simulink model "sampleModel196"  (R2021b)
settings: Solver=VariableStepAuto  StartTime=0.0  StopTime=10.0  RelTol=1e-3
undefined symbols (not defined in the file or in its folder): DiscIntNeverNeededParam
libraries: simulink x12, slpidlib x1
settings Model: Creator=user  LastModifiedBy=user

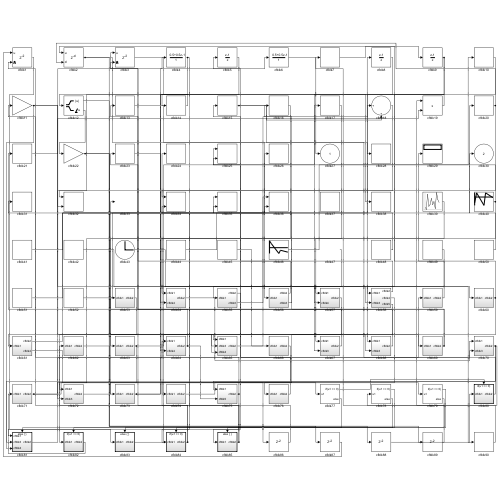
[thumbnail: Simulink's stored preview of the top-level diagram]
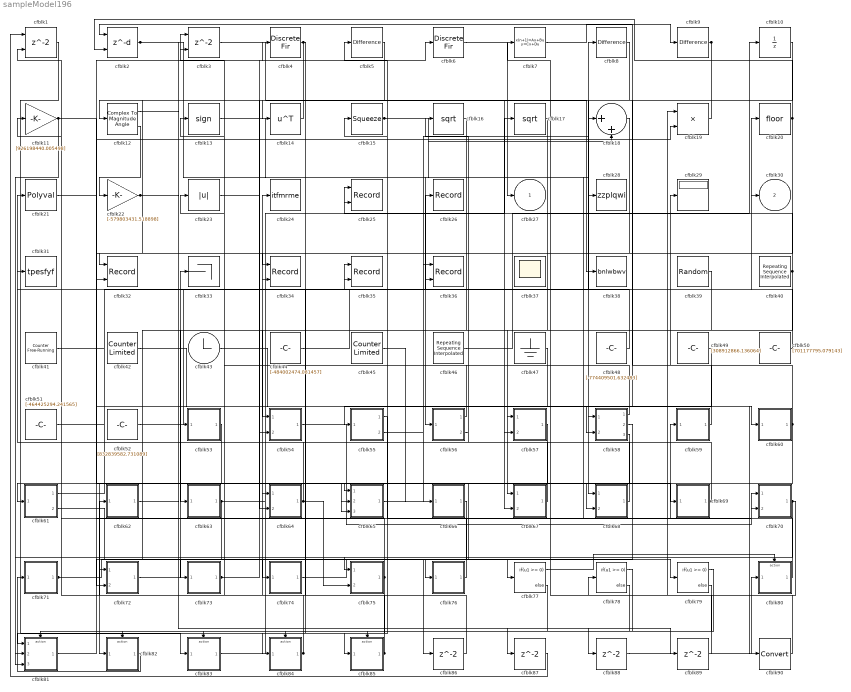
== system sampleModel196 ==
  cfblk1 : Delay  ShowEnablePort=on  SampleTime=1
      settings: InputPortMap=u0,e6
  cfblk10 : UnitDelay  HasFrameUpgradeWarning=on
  cfblk11 : Gain  Gain=[926198440.005498]
  cfblk12 : ComplexToMagnitudeAngle
  cfblk13 : Signum
  cfblk14 : Math  Operator=transpose  SaturateOnIntegerOverflow=on
  cfblk15 : Squeeze
  cfblk16 : Sqrt  SaturateOnIntegerOverflow=on
  cfblk17 : Sqrt  SaturateOnIntegerOverflow=on
  cfblk18 : Sum  Inputs=|++
  cfblk19 : Product  Inputs=**
  cfblk2 : Delay  DelayLengthSource=Input port  SampleTime=1
      settings: InputPortMap=u0,p1
  cfblk20 : Rounding
  cfblk21 : Polyval  Coefs=[ +2.081618890e-019, -1.441693666e-014, +4.719686976e-010, -8.536869453e-006, +1.621573104e-001, -8.087801117e+001 ]
  cfblk22 : Gain  Gain=[-579803431.518898]
  cfblk23 : Abs
  cfblk24 : ToWorkspace  VariableName=itfmrme  SaveFormat=Timeseries  SampleTime=-1
  cfblk25 : Record  FileSettingsInternal="{\"entries\":[{\"content\":{\"excelSettings\":{\"content\":{},\"type\":\"Streamout.ExcelSettings\"}},\"type\":\"Streamout.FileSettingStorage\",\"uuid\":\"ebd6f4a9-3581-428a-b59a-ad7a62004bd4\"}],\"packageUris\":[\"http://schema.mathworks.com/mf0/streamout_blocks/R2020a\"],\"version\":\"1.0\"}"  Layout=[1 1]  SignalsInternal="{\"entries\":[{\"content\":{\"signals\":[{\"content\":{\"blockPath\":[\"sampleModel196/cfblk25\"],\"channel\":[],\"dimensions\":[1],\"domain\":\"sampleModel196/cfblk25\",\"lineColor\":\"#a2142f\",\"plots\":[1],\"port\":1,\"sid\":[\"\"],\"signalID\":7449,\"signalName\":\"cfblk56:1\"},\"type\":\"RecordBlkView.Signal\",\"uuid\":\"a9c48982-f614-47e9-af30-97d896957ff6\"},{\"content\":{\"blockPath\":[\"sampleModel196/cfblk25\"],\"channel\":[],\"dimensions\":[1],\"domain\":\"sampleModel196/cfblk25\",\"lineColor\":\"#139fff\",\"plots\":[1],\"port\":2,\"sid\":[\"\"],\"signalID\":7453,\"signalName\":\"cfblk40\"},\"type\":\"RecordBlkView.Signal\",\"uuid\":\"ad963e30-dda2-47b4-965b-ed6e8714a0d3\"}]},\"type\":\"RecordBlkView.InputSignals\",\"uuid\":\"9b194853-d7b6-4a0e-a025-6a91142790fe\"}],\"packageUris\":[\"http://schema.mathworks.com/mf0/streamout_blocks/R2020a\"],\"version\":\"1.0\"}"  VisualizationBindings="{\"xyplotplugin\":{\"info\":[{\"series\":[{\"bindingParametersList\":[{\"parameter\":\"X-Axis\",\"signalID\":7449,\"signalName\":\"cfblk56:1\"},{\"parameter\":\"Y-Axis\",\"signalID\":7453,\"signalName\":\"cfblk40\"}],\"seriesID\":12748}],\"subplotID\":1}]}}"  CompatibilityTag=XY
  cfblk26 : Record  FileSettingsInternal="{\"entries\":[{\"content\":{\"excelSettings\":{\"content\":{},\"type\":\"Streamout.ExcelSettings\"}},\"type\":\"Streamout.FileSettingStorage\",\"uuid\":\"2445aa79-1fdb-47b8-89e7-35a85b27600f\"}],\"packageUris\":[\"http://schema.mathworks.com/mf0/streamout_blocks/R2020a\"],\"version\":\"1.0\"}"  SignalsInternal="{\"entries\":[{\"content\":{\"signals\":[{\"content\":{\"blockPath\":[\"sampleModel196/cfblk26\"],\"channel\":[],\"dimensions\":[1],\"domain\":\"sampleModel196/cfblk26\",\"lineColor\":\"#ff6929\",\"plots\":[1],\"port\":1,\"sid\":[\"\"],\"signalID\":7495,\"signalName\":\"cfblk41\"},\"type\":\"RecordBlkView.Signal\",\"uuid\":\"b33c4b9a-08ec-4f33-ba24-e1cc10466944\"}]},\"type\":\"RecordBlkView.InputSignals\",\"uuid\":\"3c88b68e-3c23-4d2f-858d-3a9c6e306d4d\"}],\"packageUris\":[\"http://schema.mathworks.com/mf0/streamout_blocks/R2020a\"],\"version\":\"1.0\"}"  VisualizationBindings="{\"sparklinesplugin\":{\"info\":[{\"bindingParametersList\":[],\"subplotID\":1}]}}"
  cfblk28 : ToWorkspace  VariableName=zzplqwi  SaveFormat=Timeseries  SampleTime=-1
  cfblk29 : Display
  cfblk3 : Delay  ShowEnablePort=on  SampleTime=1
      settings: InputPortMap=u0,e6
  cfblk31 : ToWorkspace  VariableName=tpesfyf  SaveFormat=Timeseries  SampleTime=-1
  cfblk32 : Record  FileSettingsInternal="{\"entries\":[{\"content\":{\"excelSettings\":{\"content\":{},\"type\":\"Streamout.ExcelSettings\"}},\"type\":\"Streamout.FileSettingStorage\",\"uuid\":\"bf744f18-d074-43f9-bec1-89a481855710\"}],\"packageUris\":[\"http://schema.mathworks.com/mf0/streamout_blocks/R2020a\"],\"version\":\"1.0\"}"  Layout=[1 1]  SignalsInternal="{\"entries\":[{\"content\":{\"signals\":[{\"content\":{\"blockPath\":[\"sampleModel196/cfblk32\"],\"channel\":[],\"dimensions\":[1],\"domain\":\"sampleModel196/cfblk32\",\"lineColor\":\"#a2142f\",\"plots\":[1],\"port\":1,\"sid\":[\"\"],\"signalID\":7457,\"signalName\":\"cfblk5\"},\"type\":\"RecordBlkView.Signal\",\"uuid\":\"31689776-47fe-422e-aca7-1eb21403d129\"},{\"content\":{\"blockPath\":[\"sampleModel196/cfblk32\"],\"channel\":[],\"dimensions\":[1],\"domain\":\"sampleModel196/cfblk32\",\"lineColor\":\"#139fff\",\"plots\":[1],\"port\":2,\"sid\":[\"\"],\"signalID\":7461,\"signalName\":\"cfblk20\"},\"type\":\"RecordBlkView.Signal\",\"uuid\":\"17bd4d18-57bb-470c-9e43-fdcf53ad759b\"}]},\"type\":\"RecordBlkView.InputSignals\",\"uuid\":\"335cb6c9-9546-4695-8874-e885ee878550\"}],\"packageUris\":[\"http://schema.mathworks.com/mf0/streamout_blocks/R2020a\"],\"version\":\"1.0\"}"  VisualizationBindings="{\"xyplotplugin\":{\"info\":[{\"series\":[{\"bindingParametersList\":[{\"parameter\":\"X-Axis\",\"signalID\":7457,\"signalName\":\"cfblk5\"},{\"parameter\":\"Y-Axis\",\"signalID\":7461,\"signalName\":\"cfblk20\"}],\"seriesID\":42470}],\"subplotID\":1}]}}"  CompatibilityTag=XY
  cfblk33 : Terminator
  cfblk34 : Record  FileSettingsInternal="{\"entries\":[{\"content\":{\"excelSettings\":{\"content\":{},\"type\":\"Streamout.ExcelSettings\"}},\"type\":\"Streamout.FileSettingStorage\",\"uuid\":\"44b56a1a-1e95-409d-987e-e733322c070c\"}],\"packageUris\":[\"http://schema.mathworks.com/mf0/streamout_blocks/R2020a\"],\"version\":\"1.0\"}"  Layout=[1 1]  SignalsInternal="{\"entries\":[{\"content\":{\"signals\":[{\"content\":{\"blockPath\":[\"sampleModel196/cfblk34\"],\"channel\":[],\"dimensions\":[1],\"domain\":\"sampleModel196/cfblk34\",\"lineColor\":\"#a2142f\",\"plots\":[1],\"port\":1,\"sid\":[\"\"],\"signalID\":7465,\"signalName\":\"cfblk18\"},\"type\":\"RecordBlkView.Signal\",\"uuid\":\"0f9eff3a-cfcd-403f-aa3d-d8cbb3cc7e76\"},{\"content\":{\"blockPath\":[\"sampleModel196/cfblk34\"],\"channel\":[],\"dimensions\":[1],\"domain\":\"sampleModel196/cfblk34\",\"lineColor\":\"#139fff\",\"plots\":[1],\"port\":2,\"sid\":[\"\"],\"signalID\":7469,\"signalName\":\"cfblk85\"},\"type\":\"RecordBlkView.Signal\",\"uuid\":\"d6eda2cf-49ef-4ee1-b244-38dc2486a214\"}]},\"type\":\"RecordBlkView.InputSignals\",\"uuid\":\"cf33cff3-aab6-408d-8b77-f2d2e822a3f0\"}],\"packageUris\":[\"http://schema.mathworks.com/mf0/streamout_blocks/R2020a\"],\"version\":\"1.0\"}"  VisualizationBindings="{\"xyplotplugin\":{\"info\":[{\"series\":[{\"bindingParametersList\":[{\"parameter\":\"X-Axis\",\"signalID\":7465,\"signalName\":\"cfblk18\"},{\"parameter\":\"Y-Axis\",\"signalID\":7469,\"signalName\":\"cfblk85\"}],\"seriesID\":17726}],\"subplotID\":1}]}}"  CompatibilityTag=XY
  cfblk35 : Record  FileSettingsInternal="{\"entries\":[{\"content\":{\"excelSettings\":{\"content\":{},\"type\":\"Streamout.ExcelSettings\"}},\"type\":\"Streamout.FileSettingStorage\",\"uuid\":\"7f9abc0e-2cc1-4510-b0e6-42d033897b2e\"}],\"packageUris\":[\"http://schema.mathworks.com/mf0/streamout_blocks/R2020a\"],\"version\":\"1.0\"}"  Layout=[1 1]  SignalsInternal="{\"entries\":[{\"content\":{\"signals\":[{\"content\":{\"blockPath\":[\"sampleModel196/cfblk35\"],\"channel\":[],\"dimensions\":[1],\"domain\":\"sampleModel196/cfblk35\",\"lineColor\":\"#a2142f\",\"plots\":[1],\"port\":1,\"sid\":[\"\"],\"signalID\":7473,\"signalName\":\"cfblk52\"},\"type\":\"RecordBlkView.Signal\",\"uuid\":\"3c653f7d-91cd-4ce5-b0bf-04fb68007592\"},{\"content\":{\"blockPath\":[\"sampleModel196/cfblk35\"],\"channel\":[],\"dimensions\":[1],\"domain\":\"sampleModel196/cfblk35\",\"lineColor\":\"#139fff\",\"plots\":[1],\"port\":2,\"sid\":[\"\"],\"signalID\":7477,\"signalName\":\"cfblk56:2\"},\"type\":\"RecordBlkView.Signal\",\"uuid\":\"6a33e96c-9fe5-4313-b026-49fc6d793e83\"}]},\"type\":\"RecordBlkView.InputSignals\",\"uuid\":\"7a80ccfb-8ce4-455d-850f-91369f2529a9\"}],\"packageUris\":[\"http://schema.mathworks.com/mf0/streamout_blocks/R2020a\"],\"version\":\"1.0\"}"  VisualizationBindings="{\"xyplotplugin\":{\"info\":[{\"series\":[{\"bindingParametersList\":[{\"parameter\":\"X-Axis\",\"signalID\":7473,\"signalName\":\"cfblk52\"},{\"parameter\":\"Y-Axis\",\"signalID\":7477,\"signalName\":\"cfblk56:2\"}],\"seriesID\":7674}],\"subplotID\":1}]}}"  CompatibilityTag=XY
  cfblk36 : Record  FileSettingsInternal="{\"entries\":[{\"content\":{\"excelSettings\":{\"content\":{},\"type\":\"Streamout.ExcelSettings\"}},\"type\":\"Streamout.FileSettingStorage\",\"uuid\":\"f043a9ff-7dfe-4c6c-88df-b525cd69d3e4\"}],\"packageUris\":[\"http://schema.mathworks.com/mf0/streamout_blocks/R2020a\"],\"version\":\"1.0\"}"  Layout=[1 1]  SignalsInternal="{\"entries\":[{\"content\":{\"signals\":[{\"content\":{\"blockPath\":[\"sampleModel196/cfblk36\"],\"channel\":[],\"dimensions\":[1],\"domain\":\"sampleModel196/cfblk36\",\"lineColor\":\"#a2142f\",\"plots\":[1],\"port\":1,\"sid\":[\"\"],\"signalID\":7481,\"signalName\":\"cfblk65\"},\"type\":\"RecordBlkView.Signal\",\"uuid\":\"65fcb63e-1503-467f-81bc-7a25df069058\"},{\"content\":{\"blockPath\":[\"sampleModel196/cfblk36\"],\"channel\":[],\"dimensions\":[1],\"domain\":\"sampleModel196/cfblk36\",\"lineColor\":\"#139fff\",\"plots\":[1],\"port\":2,\"sid\":[\"\"],\"signalID\":7485,\"signalName\":\"cfblk51\"},\"type\":\"RecordBlkView.Signal\",\"uuid\":\"3e54b984-48c4-4046-b527-7630b092be08\"}]},\"type\":\"RecordBlkView.InputSignals\",\"uuid\":\"370319a3-713c-4883-9ac8-89c3f3400cb0\"}],\"packageUris\":[\"http://schema.mathworks.com/mf0/streamout_blocks/R2020a\"],\"version\":\"1.0\"}"  VisualizationBindings="{\"xyplotplugin\":{\"info\":[{\"series\":[{\"bindingParametersList\":[{\"parameter\":\"X-Axis\",\"signalID\":7481,\"signalName\":\"cfblk65\"},{\"parameter\":\"Y-Axis\",\"signalID\":7485,\"signalName\":\"cfblk51\"}],\"seriesID\":38838}],\"subplotID\":1}]}}"  CompatibilityTag=XY
  cfblk37 : Scope
      settings: Floating=on
  cfblk38 : ToWorkspace  VariableName=bnlwbwv  SaveFormat=Timeseries  SampleTime=-1
  cfblk39 : UniformRandomNumber  Minimum=[-3778114337.742830]  Maximum=[8573210541.669261]  Seed=[62594337.000000]  SampleTime=0.1
  cfblk4 : DiscreteFir  SampleTime=1
  cfblk40 : simulink/Sources/Repeating Sequence Interpolated  OutValues=[-595286399.306471, 430406354.099444, -847114373.561798, 413620163.272758, -80797133.288778]  TimeValues=[0 0.1 0.5 0.6 1].'  LookUpMeth=Use Input Below  tsamp=0.01  OutMin=[]  OutMax=[]  OutDataTypeStr=double  OutputDataTypeScalingMode=double  OutDataType=fixdt(0,8)  OutScaling=2^-10
  cfblk41 : simulink/Sources/Counter Free-Running  NumBits=[48.000000]  tsamp=-1
  cfblk42 : simulink/Sources/Counter Limited  uplimit=[655.000000]  tsamp=-1
  cfblk43 : Clock
  cfblk44 : Constant  Value=[-484002474.081457]  SampleTime=1
  cfblk45 : simulink/Sources/Counter Limited  uplimit=[480.000000]  tsamp=-1
  cfblk46 : simulink/Sources/Repeating Sequence Interpolated  OutValues=[797883699.847980, 464343405.364402, -637796917.048516, -287258866.510282, -505571272.928472]  TimeValues=[0 0.1 0.5 0.6 1].'  LookUpMeth=Use Input Nearest  tsamp=0.01  OutMin=[]  OutMax=[]  OutDataTypeStr=double  OutputDataTypeScalingMode=double  OutDataType=fixdt(0,8)  OutScaling=2^-10
  cfblk47 : Ground
  cfblk48 : Constant  Value=[-774409501.632483]  SampleTime=1
  cfblk49 : Constant  Value=[308912866.136064]  SampleTime=1
  cfblk5 : simulink/Discrete/Difference  ICPrevInput=0.0  OutMin=[]  OutMax=[]  OutDataTypeStr=Inherit: Inherit via back propagation  OutDataType=fixdt(1, 16)  OutScaling=2^-10  DoSatur=off
  cfblk50 : Constant  Value=[701177795.079143]  SampleTime=1
  cfblk51 : Constant  Value=[-464425294.241565]  SampleTime=1
  cfblk52 : Constant  Value=[832839582.731089]  SampleTime=1
  cfblk53 : Subsystem
  cfblk54 : Subsystem
  cfblk55 : Subsystem
  cfblk56 : Subsystem
  cfblk57 : Subsystem
  cfblk58 : Subsystem
  cfblk59 : Subsystem
  cfblk6 : DiscreteFir  SampleTime=1
  cfblk60 : Subsystem
  cfblk61 : Subsystem
  cfblk62 : Subsystem
  cfblk63 : Subsystem
  cfblk64 : Subsystem
  cfblk65 : Subsystem
  cfblk66 : Subsystem
  cfblk67 : Subsystem
  cfblk68 : Subsystem
  cfblk69 : Subsystem
  cfblk7 : DiscreteStateSpace
  cfblk70 : Subsystem
  cfblk71 : Subsystem
  cfblk72 : Subsystem
  cfblk73 : Subsystem
  cfblk74 : Subsystem
  cfblk75 : Subsystem
  cfblk76 : Subsystem
  cfblk77 : If  IfExpression=u1 >= 0  SampleTime=1
  cfblk78 : If  IfExpression=u1 >= 0  SampleTime=1
  cfblk79 : If  IfExpression=u1 >= 0  SampleTime=1
  cfblk8 : simulink/Discrete/Difference  ICPrevInput=0.0  OutMin=[]  OutMax=[]  OutDataTypeStr=Inherit: Inherit via back propagation  OutDataType=fixdt(1, 16)  OutScaling=2^-10  DoSatur=off
  cfblk80 : Subsystem  TreatAsAtomicUnit=on
  cfblk81 : Subsystem  TreatAsAtomicUnit=on
  cfblk82 : Subsystem  TreatAsAtomicUnit=on
  cfblk83 : Subsystem  TreatAsAtomicUnit=on
  cfblk84 : Subsystem  TreatAsAtomicUnit=on
  cfblk85 : Subsystem  TreatAsAtomicUnit=on
  cfblk{86..89} (4 alike) : Delay  SampleTime=1
  cfblk9 : simulink/Discrete/Difference  ICPrevInput=0.0  OutMin=[]  OutMax=[]  OutDataTypeStr=Inherit: Inherit via back propagation  OutDataType=fixdt(1, 16)  OutScaling=2^-10  DoSatur=off
  cfblk90 : DataTypeConversion
  cfblk27 : Outport
  cfblk30 : Outport  Port=2
  wires:
  cfblk8/1 -> cfblk68/1(cfblk1)
  cfblk84/1(cfblk2) -> cfblk24/1, cfblk53/1(cfblk1)
  cfblk60/1(cfblk2) -> cfblk2/1, cfblk65/2(cfblk3)
  cfblk2/1 -> cfblk59/1(cfblk1), cfblk65/3(cfblk4)
  cfblk45/1 -> cfblk66/1(cfblk1)
  cfblk61/1(cfblk2) -> cfblk8/1
  cfblk13/1 -> cfblk56/1(cfblk1)
  cfblk41/1 -> cfblk26/1
  cfblk52/1 -> cfblk35/1
  cfblk70/1(cfblk2) -> cfblk78/1, cfblk81/3(cfblk4), cfblk75/1(cfblk1)
  cfblk20/1 -> cfblk2/2, cfblk32/2
  cfblk14/1 -> cfblk12/1
  cfblk6/1 -> cfblk27/1
  cfblk65/1(cfblk2) -> cfblk36/1
  cfblk72/1(cfblk2) -> cfblk33/1
  cfblk17/1 -> cfblk67/1(cfblk1)
  cfblk1/1 -> cfblk83/1(cfblk1)
  cfblk23/1 -> cfblk57/1(cfblk1)
  cfblk82/1(cfblk2) -> cfblk71/1(cfblk1)
  cfblk15/1 -> cfblk28/1, cfblk18/2
  cfblk83/1(cfblk2) -> cfblk17/1
  cfblk54/1(cfblk2) -> cfblk70/1(cfblk1)
  cfblk50/1 -> cfblk20/1
  cfblk51/1 -> cfblk36/2
  cfblk19/1 -> cfblk14/1
  cfblk69/1(cfblk2) -> cfblk13/1, cfblk16/1
  cfblk10/1 -> cfblk67/2(cfblk3)
  cfblk12/2 -> cfblk22/1
  cfblk57/1(cfblk2) -> cfblk82/1(cfblk1)
  cfblk46/1 -> cfblk10/1
  cfblk4/1 -> cfblk74/1(cfblk1), cfblk64/2(cfblk4)
  cfblk56/1(cfblk2) -> cfblk25/1
  cfblk58/1(cfblk2) -> cfblk23/1
  cfblk71/1(cfblk2) -> cfblk77/1, cfblk64/1(cfblk1)
  cfblk66/1(cfblk2) -> cfblk84/1(cfblk1)
  cfblk16/1 -> cfblk54/1(cfblk1)
  cfblk85/1(cfblk2) -> cfblk62/1(cfblk1), cfblk34/2
  cfblk73/1(cfblk2) -> cfblk6/1, cfblk70/2(cfblk3)
  cfblk47/1 -> cfblk55/1(cfblk1)
  cfblk53/1(cfblk2) -> cfblk61/1(cfblk1)
  cfblk75/1(cfblk2) -> cfblk81/1(cfblk1), cfblk11/1
  cfblk49/1 -> cfblk57/2(cfblk4)
  cfblk22/1 -> cfblk68/2(cfblk3), cfblk89/1
  cfblk18/1 -> cfblk34/1
  cfblk3/1 -> cfblk38/1
  cfblk74/1(cfblk2) -> cfblk79/1
  cfblk44/1 -> cfblk30/1
  cfblk55/1(cfblk2) -> cfblk85/1(cfblk1)
  cfblk21/1 -> cfblk4/1
  cfblk5/1 -> cfblk32/1
  cfblk40/1 -> cfblk72/1(cfblk1), cfblk25/2
  cfblk76/1(cfblk2) -> cfblk15/1
  cfblk59/1(cfblk2) -> cfblk29/1
  cfblk68/1(cfblk2) -> cfblk3/1
  cfblk39/1 -> cfblk63/1(cfblk1)
  cfblk7/1 -> cfblk9/1
  cfblk63/1(cfblk2) -> cfblk73/1(cfblk1), cfblk69/1(cfblk1)
  cfblk55/2(cfblk3) -> cfblk18/1
  cfblk9/1 -> cfblk58/1(cfblk1), cfblk54/2(cfblk4)
  cfblk58/2(cfblk4) -> cfblk72/2(cfblk3)
  cfblk81/1(cfblk2) -> cfblk19/2
  cfblk80/1(cfblk2) -> cfblk5/1
  cfblk67/1(cfblk2) -> cfblk21/1
  cfblk43/1 -> cfblk58/2(cfblk3)
  cfblk48/1 -> cfblk31/1
  cfblk58/3(cfblk5) -> cfblk76/1(cfblk1)
  cfblk64/1(cfblk2) -> cfblk3/2, cfblk75/2(cfblk5)
  cfblk11/1 -> cfblk81/2(cfblk3), cfblk65/1(cfblk1), cfblk60/1(cfblk1)
  cfblk56/2(cfblk3) -> cfblk35/2
  cfblk77/1 -> cfblk80/Action
  cfblk77/2 -> cfblk81/Action
  cfblk78/1 -> cfblk82/Action
  cfblk78/2 -> cfblk83/Action
  cfblk79/1 -> cfblk84/Action
  cfblk79/2 -> cfblk85/Action
  cfblk61/2(cfblk4) -> cfblk86/1
  cfblk86/1 -> cfblk1/2
  cfblk62/1(cfblk2) -> cfblk87/1
  cfblk87/1 -> cfblk1/1
  cfblk12/1 -> cfblk88/1
  cfblk88/1 -> cfblk80/1(cfblk1)
  cfblk89/1 -> cfblk19/1
  cfblk42/1 -> cfblk90/1
  cfblk90/1 -> cfblk7/1

== system sampleModel196/cfblk53 ==
  cfblk1 : Inport
  cfblk3 : Squeeze
  cfblk2 : Outport
  wires:
  cfblk1/1 -> cfblk3/1
  cfblk3/1 -> cfblk2/1

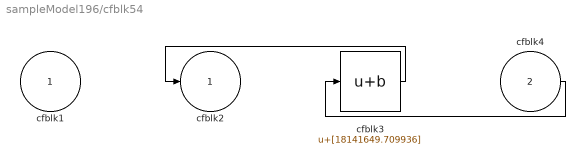
== system sampleModel196/cfblk54 ==
  cfblk1 : Inport
  cfblk4 : Inport  Port=2
  cfblk3 : Bias  Bias=[18141649.709936]
  cfblk2 : Outport
  wires:
  cfblk3/1 -> cfblk2/1
  cfblk4/1 -> cfblk3/1

== system sampleModel196/cfblk55 ==
  cfblk1 : Inport
  cfblk2 : Outport
  cfblk3 : Outport  Port=2
  wires:
  cfblk1/1 -> cfblk3/1, cfblk2/1

== system sampleModel196/cfblk56 ==
  cfblk1 : Inport
  cfblk2 : Outport
  cfblk3 : Outport  Port=2
  wires:
  cfblk1/1 -> cfblk2/1, cfblk3/1

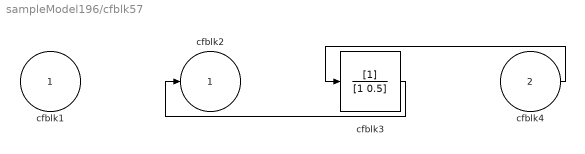
== system sampleModel196/cfblk57 ==
  cfblk1 : Inport
  cfblk4 : Inport  Port=2
  cfblk3 : DiscreteFilter  SampleTime=1
  cfblk2 : Outport
  wires:
  cfblk4/1 -> cfblk3/1
  cfblk3/1 -> cfblk2/1

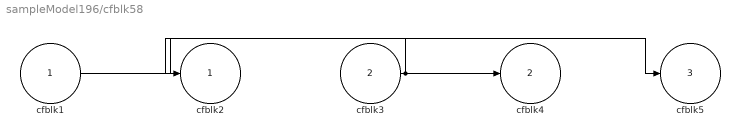
== system sampleModel196/cfblk58 ==
  cfblk1 : Inport
  cfblk3 : Inport  Port=2
  cfblk2 : Outport
  cfblk4 : Outport  Port=2
  cfblk5 : Outport  Port=3
  wires:
  cfblk3/1 -> cfblk4/1, cfblk2/1
  cfblk1/1 -> cfblk5/1

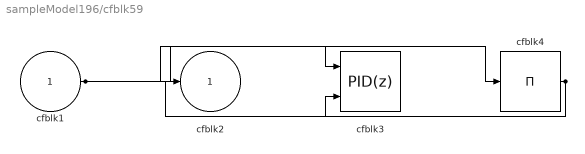
== system sampleModel196/cfblk59 ==
  cfblk1 : Inport
  cfblk3 : slpidlib/PID Controller (2DOF)  Controller=PID  Form=Parallel  TimeDomain=Discrete-time  UseExternalTs=off  SampleTime=1  IntegratorMethod=Forward Euler  FilterMethod=Forward Euler  ControllerParametersSource=internal  P=1  I=1  D=0  UseFilter=on  N=100  b=1  c=1  TunerSelectOption=Transfer Function Based (PID Tuner App)  InitialConditionSource=internal  InitialConditionForIntegrator=0  InitialConditionForFilter=0  DifferentiatorICPrevScaledInput=0  ExternalReset=none  TrackingMode=off  Kt=1  LimitOutput=off  SatLimitsSource=internal  UpperSaturationLimit=inf  LowerSaturationLimit=-inf  LinearizeAsGain=off  AntiWindupMode=none  Kb=1  POutMin=[]  POutMax=[]  IOutMin=[]  IOutMax=[]  DOutMin=[]  DOutMax=[]  NOutMin=[]  NOutMax=[]  bOutMin=[]  bOutMax=[]  cOutMin=[]  cOutMax=[]  SumOutMin=[]  SumOutMax=[]  SaturationOutMin=[]  SaturationOutMax=[]  PParamMin=[]  PParamMax=[]  IParamMin=[]  IParamMax=[]  DParamMin=[]  DParamMax=[]  NParamMin=[]  NParamMax=[]  bParamMin=[]  bParamMax=[]  cParamMin=[]  cParamMax=[]  KbParamMin=[]  KbParamMax=[]  KtParamMin=[]  KtParamMax=[]  KbOutMin=[]  KbOutMax=[]  KtOutMin=[]  KtOutMax=[]  IntegratorOutMin=[]  IntegratorOutMax=[]  FilterOutMin=[]  FilterOutMax=[]  SumI1OutMin=[]  SumI1OutMax=[]  SumI2OutMin=[]  SumI2OutMax=[]  SumI3OutMin=[]  SumI3OutMax=[]  SumI4OutMin=[]  SumI4OutMax=[]  SumDOutMin=[]  SumDOutMax=[]  Sum1OutMin=[]  Sum1OutMax=[]  Sum2OutMin=[]  Sum2OutMax=[]  Sum3OutMin=[]  Sum3OutMax=[]  DifferentiatorOutMin=[]  DifferentiatorOutMax=[]  FilterDiffOutCoefMin=[]  FilterDiffOutCoefMax=[]  ReciprocalOutMin=[]  ReciprocalOutMax=[]  SumDenOutMin=[]  SumDenOutMax=[]  SumNumOutMin=[]  SumNumOutMax=[]  DivideOutMin=[]  DivideOutMax=[]  UdiffTsProdOutMin=[]  UdiffTsProdOutMax=[]  NTsProdOutMin=[]  NTsProdOutMax=[]  UintegralTsProdOutMin=[]  UintegralTsProdOutMax=[]  UngainTsProdOutMin=[]  UngainTsProdOutMax=[]  IntegratorContinuousStateAttributes=''  IntegratorStateMustResolveToSignalObject=off  IntegratorRTWStateStorageClass=Auto  FilterContinuousStateAttributes=''  FilterStateMustResolveToSignalObject=off  FilterRTWStateStorageClass=Auto  ParallelPVariant=InternalParameters  IdealPVariant=Disabled  IVariant=InternalParameters  DVariant=InternalParameters  bVariant=InternalParameters  cVariant=InternalParameters  IntegratorVariant=Discrete  SatVariant=Disabled  AWVariant=Passthrough  PCopyVariant=Disabled  TRVariant=Disabled  FdbkBlocksVariant=Forward  IdealPFdbkVariant=Disabled  SatFdbkVariant=Disabled  DerivativeFilterVariant=ForwardEulerFilter  NVariant=InternalParameters  NCopyVariant=Disabled  FilterICVariant=InternalICsFilter  IntegratorICVariant=InternalICs  ExternalResetVariant=Disabled  TRSumVariant=Passthrough  SumFdbkVariant=Disabled  SumVariant=Sum_PID  TsampFilterVariant=InternalTs  TsampNgainVariant=Passthrough  TsampIntegralVariant=Passthrough  ExternalSaturationOutDataTypeStr=Inherit: Same as second input
      settings: SourceProductBaseCode=SL
  cfblk4 : Product  Inputs=*
  cfblk2 : Outport
  wires:
  cfblk1/1 -> cfblk4/1, cfblk3/1
  cfblk4/1 -> cfblk2/1, cfblk3/2

== system sampleModel196/cfblk60 ==
  cfblk1 : Inport
  cfblk3 : simulink/Discrete/Transfer Fcn Real Zero  ZeroZ=0.75  ICPrevInput=0.0  DoSatur=off
      settings: SourceProductBaseCode=SL
  cfblk4 : Assignment  DiagnosticForDimensions=Warning  IndexOptions=Index vector (dialog)  Indices=1  OutputSizes=1
  cfblk2 : Outport
  wires:
  cfblk1/1 -> cfblk3/1, cfblk4/2
  cfblk3/1 -> cfblk2/1, cfblk4/1

== system sampleModel196/cfblk61 ==
  cfblk1 : Inport
  cfblk3 : simulink/Discrete/Transfer Fcn Real Zero  ZeroZ=0.75  ICPrevInput=0.0  DoSatur=off
      settings: SourceProductBaseCode=SL
  cfblk2 : Outport
  cfblk4 : Outport  Port=2
  wires:
  cfblk1/1 -> cfblk2/1, cfblk3/1
  cfblk3/1 -> cfblk4/1

== system sampleModel196/cfblk62 ==
  cfblk1 : Inport
  cfblk3 : Math  Operator=conj  SaturateOnIntegerOverflow=on
  cfblk2 : Outport
  wires:
  cfblk1/1 -> cfblk2/1, cfblk3/1

== system sampleModel196/cfblk63 ==
  cfblk1 : Inport
  cfblk3 : Product  Inputs=**
  cfblk2 : Outport
  wires:
  cfblk3/1 -> cfblk2/1
  cfblk1/1 -> cfblk3/1, cfblk3/2

== system sampleModel196/cfblk64 ==
  cfblk1 : Inport
  cfblk4 : Inport  Port=2
  cfblk3 : Gain  Gain=[-609765210.525331]
  cfblk2 : Outport
  wires:
  cfblk1/1 -> cfblk3/1
  cfblk4/1 -> cfblk2/1

== system sampleModel196/cfblk65 ==
  cfblk1 : Inport
  cfblk3 : Inport  Port=2
  cfblk4 : Inport  Port=3
  cfblk2 : Outport
  wires:
  cfblk3/1 -> cfblk2/1

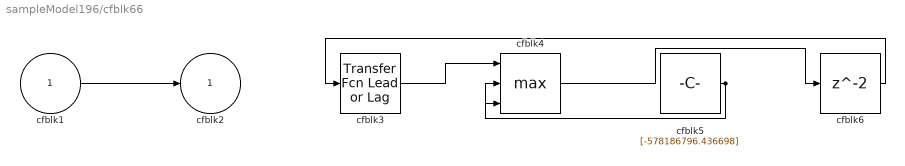
== system sampleModel196/cfblk66 ==
  cfblk1 : Inport
  cfblk3 : simulink/Discrete/Transfer Fcn Lead or Lag  PoleZ=0.95  ZeroZ=0.75  ICPrevOutput=0.0  ICPrevInput=0.0  DoSatur=off
      settings: SourceProductBaseCode=SL
  cfblk4 : MinMax  Function=max  Inputs=3
  cfblk5 : Constant  Value=[-578186796.436698]  SampleTime=1
  cfblk6 : Delay  SampleTime=1
  cfblk2 : Outport
  wires:
  cfblk1/1 -> cfblk2/1
  cfblk3/1 -> cfblk4/1
  cfblk5/1 -> cfblk4/2, cfblk4/3
  cfblk4/1 -> cfblk6/1
  cfblk6/1 -> cfblk3/1

== system sampleModel196/cfblk67 ==
  cfblk1 : Inport
  cfblk3 : Inport  Port=2
  cfblk2 : Outport
  wires:
  cfblk1/1 -> cfblk2/1

== system sampleModel196/cfblk68 ==
  cfblk1 : Inport
  cfblk3 : Inport  Port=2
  cfblk2 : Outport
  wires:
  cfblk3/1 -> cfblk2/1

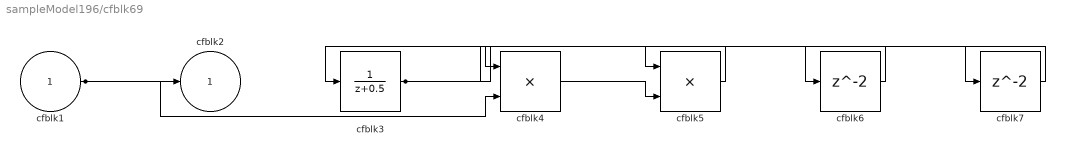
== system sampleModel196/cfblk69 ==
  cfblk1 : Inport
  cfblk3 : DiscreteTransferFcn  SampleTime=1
  cfblk4 : Product
  cfblk5 : Product  Inputs=**
  cfblk6 : Delay  SampleTime=1
  cfblk7 : Delay  SampleTime=1
  cfblk2 : Outport
  wires:
  cfblk1/1 -> cfblk2/1, cfblk4/2
  cfblk5/1 -> cfblk3/1
  cfblk3/1 -> cfblk6/1, cfblk7/1
  cfblk4/1 -> cfblk5/2
  cfblk6/1 -> cfblk5/1
  cfblk7/1 -> cfblk4/1

== system sampleModel196/cfblk70 ==
  cfblk1 : Inport
  cfblk3 : Inport  Port=2
  cfblk2 : Outport
  wires:
  cfblk1/1 -> cfblk2/1

== system sampleModel196/cfblk71 ==
  cfblk1 : Inport
  cfblk3 : Product  Inputs=**
  cfblk4 : Constant  Value=[587634203.654360]  SampleTime=1
  cfblk2 : Outport
  wires:
  cfblk4/1 -> cfblk3/1
  cfblk3/1 -> cfblk2/1
  cfblk1/1 -> cfblk3/2

== system sampleModel196/cfblk72 ==
  cfblk1 : Inport
  cfblk3 : Inport  Port=2
  cfblk2 : Outport
  wires:
  cfblk1/1 -> cfblk2/1

== system sampleModel196/cfblk73 ==
  cfblk1 : Inport
  cfblk3 : Abs
  cfblk2 : Outport
  wires:
  cfblk3/1 -> cfblk2/1
  cfblk1/1 -> cfblk3/1

== system sampleModel196/cfblk74 ==
  cfblk1 : Inport
  cfblk3 : UnitDelay  HasFrameUpgradeWarning=on
  cfblk4 : Squeeze
  cfblk2 : Outport
  wires:
  cfblk1/1 -> cfblk4/1
  cfblk4/1 -> cfblk3/1
  cfblk3/1 -> cfblk2/1

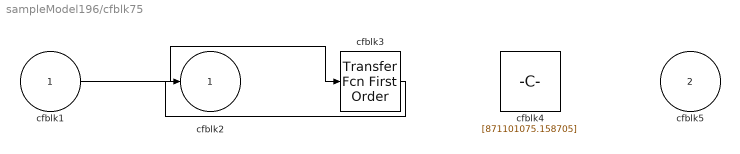
== system sampleModel196/cfblk75 ==
  cfblk1 : Inport
  cfblk5 : Inport  Port=2
  cfblk3 : simulink/Discrete/Transfer Fcn First Order  PoleZ=0.95  ICPrevOutput=0.0  DoSatur=off
  cfblk4 : Constant  Value=[871101075.158705]  SampleTime=1
  cfblk2 : Outport
  wires:
  cfblk1/1 -> cfblk3/1
  cfblk3/1 -> cfblk2/1

== system sampleModel196/cfblk76 ==
  cfblk1 : Inport
  cfblk3 : Sum  Inputs=-+
  cfblk2 : Outport
  wires:
  cfblk1/1 -> cfblk2/1, cfblk3/1, cfblk3/2

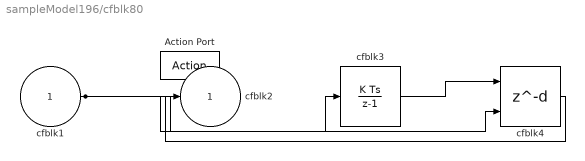
== system sampleModel196/cfblk80 ==
  cfblk1 : Inport
  Action Port : ActionPort  ActionPortLabel=if(u1 >= 0)
  cfblk3 : DiscreteIntegrator  SampleTime=-1  ICPrevOutput=DiscIntNeverNeededParam  ICPrevScaledInput=DiscIntNeverNeededParam
  cfblk4 : Delay  DelayLengthSource=Input port
      settings: InputPortMap=u0,p1
  cfblk2 : Outport
  wires:
  cfblk1/1 -> cfblk3/1, cfblk4/2
  cfblk3/1 -> cfblk4/1
  cfblk4/1 -> cfblk2/1

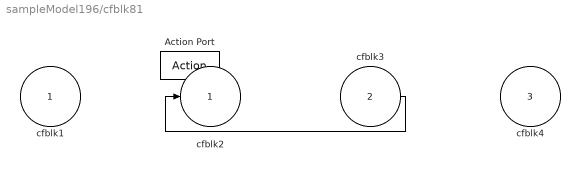
== system sampleModel196/cfblk81 ==
  cfblk1 : Inport
  cfblk3 : Inport  Port=2
  cfblk4 : Inport  Port=3
  Action Port : ActionPort  ActionPortLabel=else
  cfblk2 : Outport
  wires:
  cfblk3/1 -> cfblk2/1

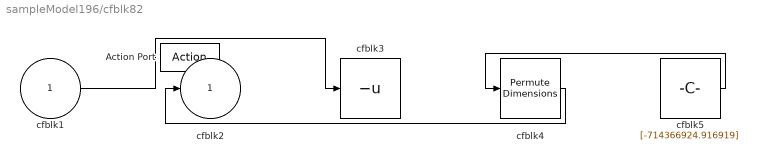
== system sampleModel196/cfblk82 ==
  cfblk1 : Inport
  Action Port : ActionPort  ActionPortLabel=if(u1 >= 0)
  cfblk3 : UnaryMinus
  cfblk4 : PermuteDimensions
  cfblk5 : Constant  Value=[-714366924.916919]  SampleTime=1
  cfblk2 : Outport
  wires:
  cfblk5/1 -> cfblk4/1
  cfblk4/1 -> cfblk2/1
  cfblk1/1 -> cfblk3/1

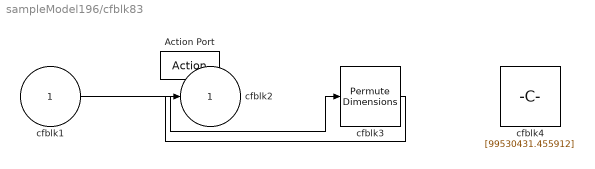
== system sampleModel196/cfblk83 ==
  cfblk1 : Inport
  Action Port : ActionPort  ActionPortLabel=else
  cfblk3 : PermuteDimensions
  cfblk4 : Constant  Value=[99530431.455912]  SampleTime=1
  cfblk2 : Outport
  wires:
  cfblk1/1 -> cfblk3/1
  cfblk3/1 -> cfblk2/1

== system sampleModel196/cfblk84 ==
  cfblk1 : Inport
  Action Port : ActionPort  ActionPortLabel=if(u1 >= 0)
  cfblk3 : UnitDelay  SampleTime=-1  HasFrameUpgradeWarning=on
  cfblk2 : Outport
  wires:
  cfblk1/1 -> cfblk3/1
  cfblk3/1 -> cfblk2/1

== system sampleModel196/cfblk85 ==
  cfblk1 : Inport
  Action Port : ActionPort  ActionPortLabel=else
  cfblk3 : Trigonometry
  cfblk2 : Outport
  wires:
  cfblk1/1 -> cfblk3/1
  cfblk3/1 -> cfblk2/1
